simulink model "Copy_of_model"  (R2016b)
settings: Solver=FixedStepAuto  StartTime=0.0  StopTime=150  FixedStep=0.01  RelTol=1e-3
undefined symbols (not defined in the file or in its folder): DiscIntNeverNeededParam
libraries: dspsrcs4 x1
settings Model: Creator=Utente  LastModifiedBy=liana

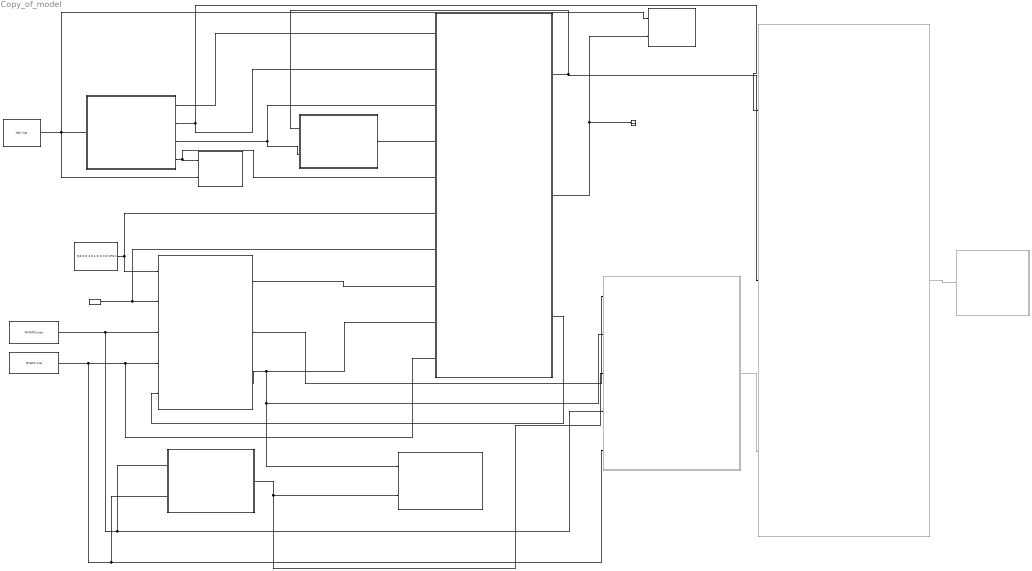
== system Copy_of_model ==
  Algebraic Transformation : Subsystem
  Attitude Observer : Subsystem
  Error position (AT) : Subsystem
  Error position (NLO) : Subsystem
  From File2 : FromFile  FileName=MYGYRO.mat  SampleTime=0.01
  From File3 : FromFile  FileName=MYACC.mat  SampleTime=0.01
  Gain computation : Subsystem
  Kalman - Bucy Filter : Subsystem  Commented=on
  Kp : Constant  Value=[10 0 0; 0 0.1 0; 0 0 0.1]*0.1  SampleTime=-1
  Mechanisation : Subsystem
  Scope : Scope
  Translational Motion Observer : Subsystem
  Vehicle position in NED : FromFile  FileName=NAV.mat
  angles error : Subsystem
  error : Subsystem  Commented=on
  sigma : Constant  Value=5  SampleTime=-1
  u computation : Subsystem  Commented=on
  wires:
  From File2/1 -> u computation/4(w_ib), Mechanisation/1(w_ib), Attitude Observer/3(w_ib)
  From File3/1 -> u computation/5(f_b), Mechanisation/2(f_b), Translational Motion Observer/10(f_b), Attitude Observer/4(f_b)
  Kp/1 -> Translational Motion Observer/6(K_p), Attitude Observer/1(Kp)
  sigma/1 -> Attitude Observer/2(sigma), Translational Motion Observer/7(sigma)
  Attitude Observer/1(J) -> Translational Motion Observer/8(J)
  Attitude Observer/3(R_nb_stim) -> angles error/1(R_nb_stim), u computation/2(R_nb_stim), Translational Motion Observer/9(R_nb_stim)
  Gain computation/1(K) -> Translational Motion Observer/4(K)
  Algebraic Transformation/3(C_dx) -> Gain computation/2(C_dx), Translational Motion Observer/3(C_dx)
  Translational Motion Observer/2(x_stim) -> Scope/1, Error position (NLO)/2(estimated)
  Vehicle position in NED/1 -> Error position (NLO)/1(true), Error position (AT)/2(true), Algebraic Transformation/1(p_n)
  Translational Motion Observer/3(f_n_stim) -> Attitude Observer/5(f_n_stim)
  Algebraic Transformation/4(x_at) -> Error position (AT)/1(estimated), Translational Motion Observer/5(Init)
  Mechanisation/1(R_nb) -> u computation/3(R_nb), angles error/2(R_nb)
  Algebraic Transformation/1(p_n_i) -> Translational Motion Observer/1(p_n_i)
  Translational Motion Observer/1(C_dx_NLO) -> Gain computation/1(C_dx_NLO), Kalman - Bucy Filter/2(C)
  Algebraic Transformation/2(delta) -> Translational Motion Observer/2(delta), Kalman - Bucy Filter/1(y)
  Attitude Observer/2(b_stim) -> u computation/1(b_stim)
  u computation/1(u) -> Kalman - Bucy Filter/3(U)
  Kalman - Bucy Filter/1(csi) -> error/1(csi)

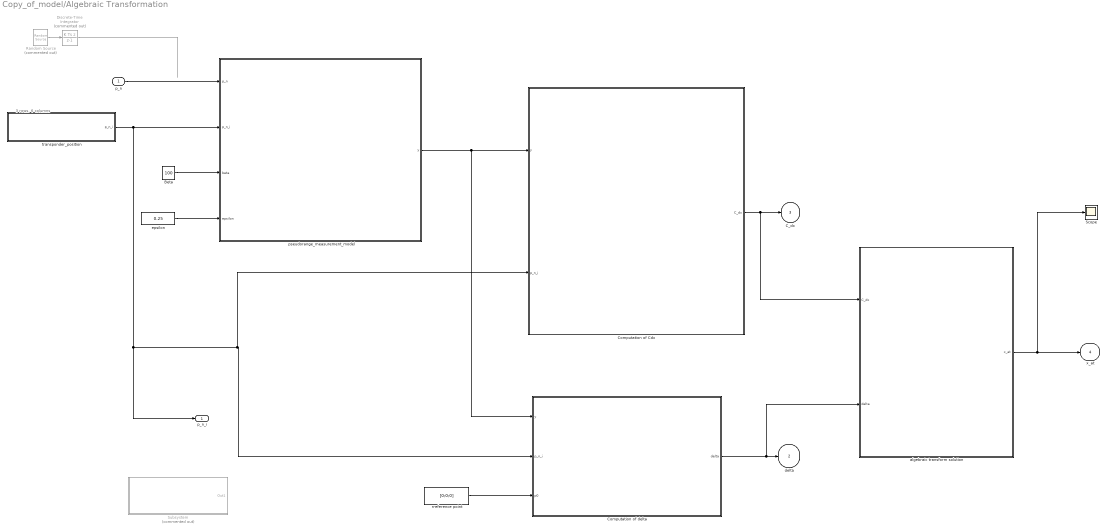
== system Copy_of_model/Algebraic Transformation ==
  note: 3 rows, 6 columns
  p_n : Inport
  Beta : Constant  Value=100
  Computation of Cdx : MATLAB Function  TreatAsAtomicUnit=on
  Computation of delta : MATLAB Function  TreatAsAtomicUnit=on
  Discrete-Time Integrator : DiscreteIntegrator  Commented=on  IntegratorMethod=Integration: Backward Euler  InitialConditionSetting=State (most efficient)  SampleTime=0.1  LimitOutput=on  UpperSaturationLimit=10  LowerSaturationLimit=-10  ICPrevOutput=DiscIntNeverNeededParam  ICPrevScaledInput=DiscIntNeverNeededParam
  Random Source : dspsrcs4/Random Source  Commented=on  SrcType=Gaussian  NormMethod=Ziggurat  CltLength=12  MinVal=0  MaxVal=1  MeanVal=[0;0;0]  VarVal=[1;1;1]*10  RepMode=Not repeatable  rawSeed=1  IsInherit=off  SampMode=Discrete  SampTime=0.1  SampFrame=1  DataType=Double  OutComplex=Real  OutputFrames=off
  Scope : Scope
  Subsystem : Subsystem  Commented=on
  algebraic transform solution : MATLAB Function  TreatAsAtomicUnit=on
  epsilon : Constant  Value=0.25
  pseudorange_measurement_model : MATLAB Function  TreatAsAtomicUnit=on
  rreference point : Constant  Value=[0;0;0]
  transponder_position : Subsystem
  p_n_i : Outport
  delta : Outport  Port=2
  C_dx : Outport  Port=3
  x_at : Outport  Port=4
  wires:
  Beta/1 -> pseudorange_measurement_model/3(beta)
  epsilon/1 -> pseudorange_measurement_model/4(epsilon)
  pseudorange_measurement_model/1(y) -> Computation of delta/1(y), Computation of Cdx/1(y)
  Computation of delta/1(delta) -> algebraic transform solution/2(delta), delta/1
  Computation of Cdx/1(C_dx) -> C_dx/1, algebraic transform solution/1(C_dx)
  rreference point/1 -> Computation of delta/3(p0)
  algebraic transform solution/1(x_at) -> Scope/1, x_at/1
  p_n/1 -> pseudorange_measurement_model/1(p_n)
  Discrete-Time Integrator/1 -> ?
  Random Source/1 -> Discrete-Time Integrator/1
  transponder_position/1(p_n_i) -> Computation of Cdx/2(p_n_i), Computation of delta/2(p_n_i), p_n_i/1, pseudorange_measurement_model/2(p_n_i)

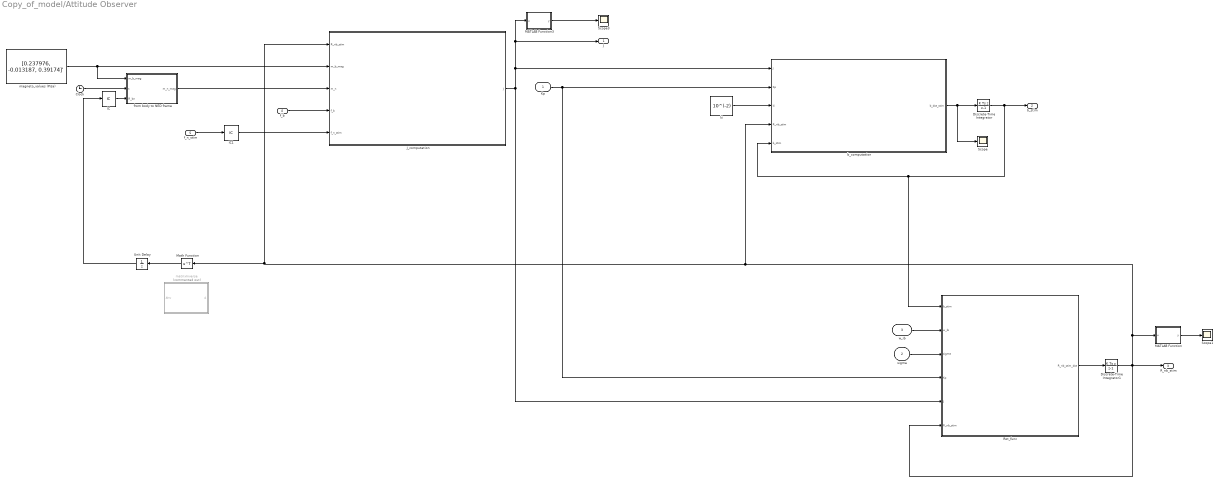
== system Copy_of_model/Attitude Observer ==
  Kp : Inport
  sigma : Inport  Port=2
  w_ib : Inport  Port=3
  f_b : Inport  Port=4
  f_n_stim : Inport  Port=5
  Clock : Clock
  Discrete-Time Integrator : DiscreteIntegrator  IntegratorMethod=Integration: Backward Euler  InitialConditionSetting=State (most efficient)  SampleTime=-1  ICPrevOutput=DiscIntNeverNeededParam  ICPrevScaledInput=DiscIntNeverNeededParam
  Discrete-Time Integrator1 : DiscreteIntegrator  IntegratorMethod=Integration: Backward Euler  InitialCondition=eye(3)  InitialConditionSetting=State (most efficient)  SampleTime=-1  ICPrevOutput=DiscIntNeverNeededParam  ICPrevScaledInput=DiscIntNeverNeededParam
  IC : InitialCondition  Value=eye(3)
  IC1 : InitialCondition  Value=[0;0;0]
  J_computation : Subsystem
  MATLAB Function : MATLAB Function  TreatAsAtomicUnit=on
  MATLAB Function3 : MATLAB Function  TreatAsAtomicUnit=on
  Math Function : Math  Operator=transpose  SaturateOnIntegerOverflow=on
  Rot_func : MATLAB Function  TreatAsAtomicUnit=on
  Scope : Scope
  Scope1 : Scope
  Scope3 : Scope
  Unit Delay : UnitDelay  SampleTime=-1
  b_computation : MATLAB Function  TreatAsAtomicUnit=on
  from body to NED frame : MATLAB Function  TreatAsAtomicUnit=on
  ki : Constant  Value=10^(-2)  SampleTime=-1
  magneto_values (Pisa) : Constant  Value=[0.237976, -0.013187, 0.39174]'
  matrixInverse : MATLAB Function  Commented=on  TreatAsAtomicUnit=on
  J : Outport
  b_stim : Outport  Port=2
  R_nb_stim : Outport  Port=3
  wires:
  magneto_values (Pisa)/1 -> from body to NED frame/1(m_b_mag), J_computation/2(m_b_mag)
  from body to NED frame/1(m_n_mag) -> J_computation/3(m_n)
  f_b/1 -> J_computation/4(f_b)
  J_computation/1(J) -> MATLAB Function3/1(u), J/1, b_computation/1(J), Rot_func/5(J)
  Kp/1 -> Rot_func/4(Kp), b_computation/2(Kp)
  ki/1 -> b_computation/3(ki)
  sigma/1 -> Rot_func/3(sigma)
  w_ib/1 -> Rot_func/2(w_ib)
  Clock/1 -> from body to NED frame/2(t)
  b_computation/1(b_dot_stim) -> Scope/1, Discrete-Time Integrator/1
  MATLAB Function/1(y) -> Scope1/1
  MATLAB Function3/1(y) -> Scope3/1
  f_n_stim/1 -> IC1/1
  Rot_func/1(R_nb_stim_dot) -> Discrete-Time Integrator1/1
  Discrete-Time Integrator/1 -> b_stim/1, Rot_func/1(b_stim), b_computation/5(b_stim)
  Discrete-Time Integrator1/1 -> R_nb_stim/1, Rot_func/6(R_nb_stim), Math Function/1, J_computation/1(R_nb_stim), b_computation/4(R_nb_stim), MATLAB Function/1(u)
  IC/1 -> from body to NED frame/3(R_bn)
  Math Function/1 -> Unit Delay/1
  Unit Delay/1 -> IC/1
  IC1/1 -> J_computation/5(f_n_stim)

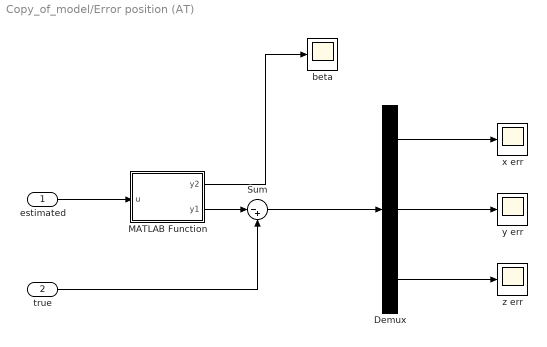
== system Copy_of_model/Error position (AT) ==
  estimated : Inport
  true : Inport  Port=2
  Demux : Demux  Outputs=3
  MATLAB Function : MATLAB Function  TreatAsAtomicUnit=on
  Sum : Sum  Inputs=|-+
  beta : Scope
  x err : Scope
  y err : Scope
  z err : Scope
  wires:
  estimated/1 -> MATLAB Function/1(u)
  MATLAB Function/2(y1) -> Sum/1
  true/1 -> Sum/2
  Sum/1 -> Demux/1
  Demux/1 -> x err/1
  Demux/2 -> y err/1
  Demux/3 -> z err/1
  MATLAB Function/1(y2) -> beta/1

== system Copy_of_model/Error position (NLO) ==
  true : Inport
  estimated : Inport  Port=2
  Demux : Demux  Outputs=3
  MATLAB Function : MATLAB Function  TreatAsAtomicUnit=on
  Sum : Sum  Inputs=|-+
  x err : Scope
  y err : Scope
  z err : Scope
  wires:
  estimated/1 -> MATLAB Function/1(u)
  MATLAB Function/1(y) -> Sum/1
  true/1 -> Sum/2
  Sum/1 -> Demux/1
  Demux/1 -> x err/1
  Demux/2 -> y err/1
  Demux/3 -> z err/1

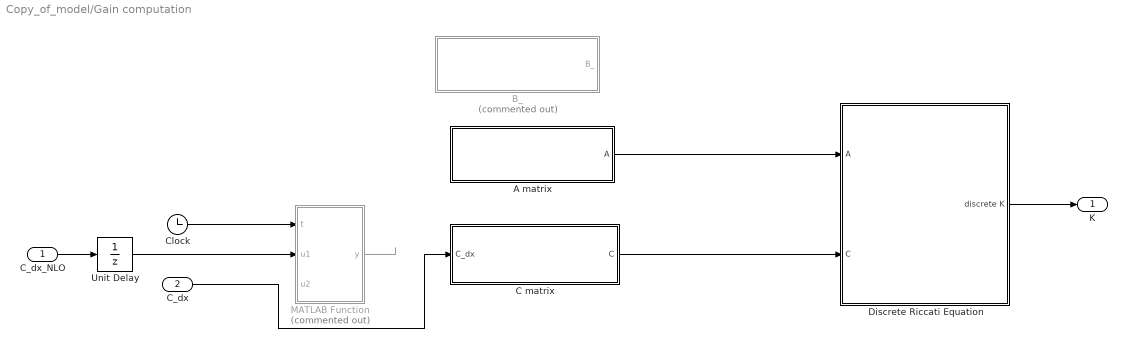
== system Copy_of_model/Gain computation ==
  C_dx_NLO : Inport
  C_dx : Inport  Port=2
  A matrix : MATLAB Function  TreatAsAtomicUnit=on
  B_ : MATLAB Function  Commented=on  TreatAsAtomicUnit=on
  C matrix : MATLAB Function  TreatAsAtomicUnit=on
  Clock : Clock
  Discrete Riccati Equation : Subsystem
  MATLAB Function : MATLAB Function  Commented=on  TreatAsAtomicUnit=on
  Unit Delay : UnitDelay  SampleTime=-1
  K : Outport
  wires:
  C matrix/1(C) -> Discrete Riccati Equation/2(C)
  A matrix/1(A) -> Discrete Riccati Equation/1("A ")
  C_dx/1 -> C matrix/1(C_dx)
  Discrete Riccati Equation/1(discrete K) -> K/1
  Clock/1 -> MATLAB Function/1(t)
  C_dx_NLO/1 -> Unit Delay/1
  MATLAB Function/1(y) -> ?
  Unit Delay/1 -> MATLAB Function/2(u1)

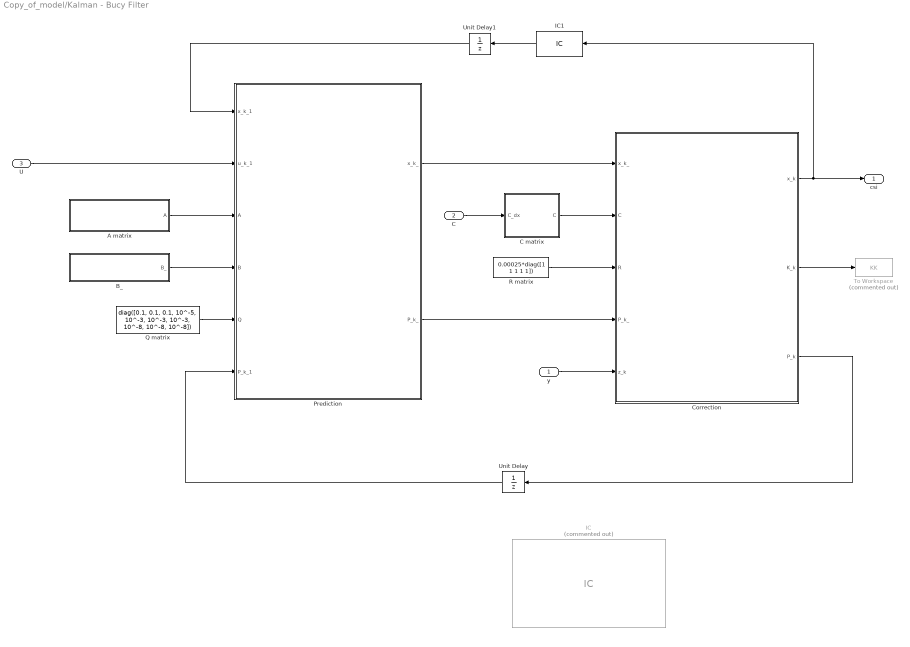
== system Copy_of_model/Kalman - Bucy Filter ==
  y : Inport
  C : Inport  Port=2
  U : Inport  Port=3
  A matrix : MATLAB Function  TreatAsAtomicUnit=on
  B_ : MATLAB Function  TreatAsAtomicUnit=on
  C matrix : MATLAB Function  TreatAsAtomicUnit=on
  Correction : MATLAB Function  TreatAsAtomicUnit=on
  IC : InitialCondition  Commented=on  Value=diag([3*(10^3),3*(10^3),3*(10^3),3*(10^3),10,10,10,0.01,0.01,0.01])
  IC1 : InitialCondition  Value=zeros(10,1)
  Prediction : MATLAB Function  TreatAsAtomicUnit=on
  Q matrix : Constant  Value=diag([0.1, 0.1, 0.1, 10^-5, 10^-3, 10^-3, 10^-3, 10^-8, 10^-8, 10^-8])
  R matrix : Constant  Value=0.00025*diag([1 1 1 1 1])
  To Workspace : ToWorkspace  Commented=on  VariableName=KK  SaveFormat=Timeseries  SampleTime=-1
  Unit Delay : UnitDelay  InitialCondition=eye(10)*10  SampleTime=-1
  Unit Delay1 : UnitDelay  SampleTime=-1
  csi : Outport
  wires:
  Prediction/2(P_k_) -> Correction/4(P_k_)
  Prediction/1(x_k_) -> Correction/1(x_k_)
  Correction/1(x_k) -> csi/1, IC1/1
  A matrix/1(A) -> Prediction/3(A)
  C matrix/1(C) -> Correction/2(C)
  B_/1(B_) -> Prediction/4(B)
  U/1 -> Prediction/2(u_k_1)
  R matrix/1 -> Correction/3(R)
  Correction/3(P_k) -> Unit Delay/1
  Unit Delay/1 -> Prediction/6(P_k_1)
  Correction/2(K_k) -> To Workspace/1
  Unit Delay1/1 -> Prediction/1(x_k_1)
  y/1 -> Correction/5(z_k)
  Q matrix/1 -> Prediction/5(Q)
  IC1/1 -> Unit Delay1/1
  C/1 -> C matrix/1(C_dx)

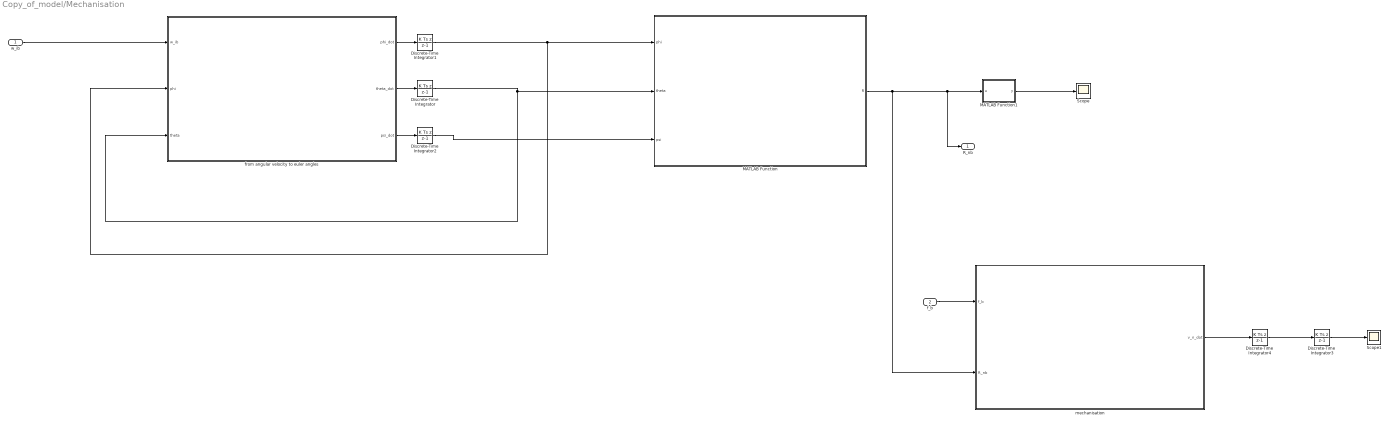
== system Copy_of_model/Mechanisation ==
  w_ib : Inport
  f_b : Inport  Port=2
  Discrete-Time Integrator{,1..4} (5 alike) : DiscreteIntegrator  IntegratorMethod=Integration: Backward Euler  InitialConditionSetting=State (most efficient)  SampleTime=-1  ICPrevOutput=DiscIntNeverNeededParam  ICPrevScaledInput=DiscIntNeverNeededParam
  MATLAB Function : MATLAB Function  TreatAsAtomicUnit=on
  MATLAB Function1 : MATLAB Function  TreatAsAtomicUnit=on
  Scope : Scope
  Scope1 : Scope
  from angular velocity to euler angles : MATLAB Function  TreatAsAtomicUnit=on
  mechanisation : MATLAB Function  TreatAsAtomicUnit=on
  R_nb : Outport
  wires:
  w_ib/1 -> from angular velocity to euler angles/1(w_ib)
  from angular velocity to euler angles/1(phi_dot) -> Discrete-Time Integrator1/1
  from angular velocity to euler angles/2(theta_dot) -> Discrete-Time Integrator/1
  from angular velocity to euler angles/3(psi_dot) -> Discrete-Time Integrator2/1
  MATLAB Function/1(R) -> mechanisation/2(R_nb), R_nb/1, MATLAB Function1/1(u)
  MATLAB Function1/1(y) -> Scope/1
  f_b/1 -> mechanisation/1(f_b)
  Discrete-Time Integrator4/1 -> Discrete-Time Integrator3/1
  Discrete-Time Integrator3/1 -> Scope1/1
  mechanisation/1(v_n_dot) -> Discrete-Time Integrator4/1
  Discrete-Time Integrator/1 -> from angular velocity to euler angles/3(theta), MATLAB Function/2(theta)
  Discrete-Time Integrator2/1 -> MATLAB Function/3(psi)
  Discrete-Time Integrator1/1 -> from angular velocity to euler angles/2(phi), MATLAB Function/1(phi)

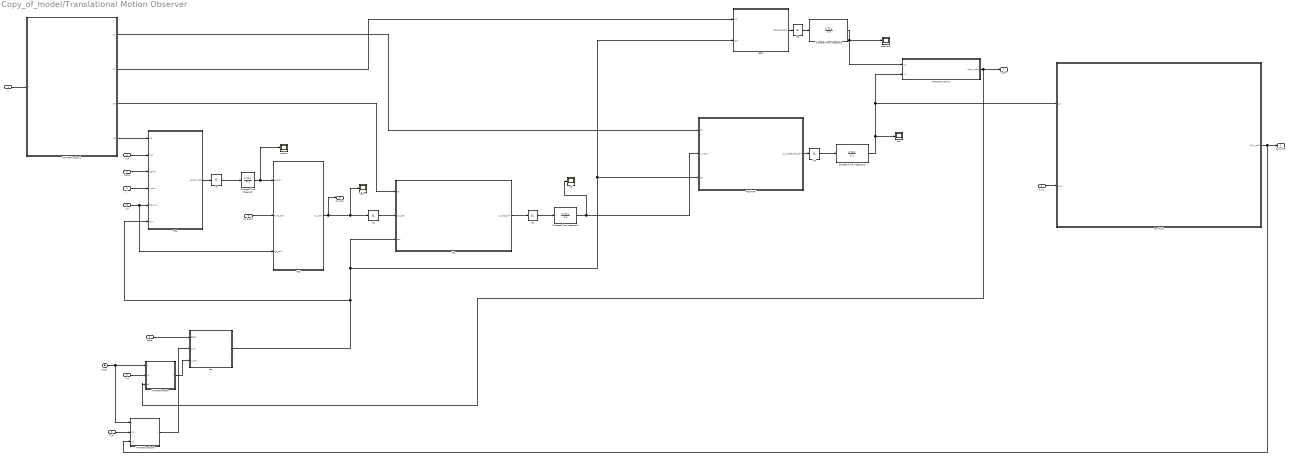
== system Copy_of_model/Translational Motion Observer ==
  p_n_i : Inport
  delta : Inport  Port=2
  C_dx : Inport  Port=3
  K : Inport  Port=4
  Init : Inport  Port=5
  K_p : Inport  Port=6
  sigma : Inport  Port=7
  J : Inport  Port=8
  R_nb_stim : Inport  Port=9
  f_b : Inport  Port=10
  ACC : MATLAB Function  TreatAsAtomicUnit=on
  BETA : MATLAB Function  TreatAsAtomicUnit=on
  Clock : Clock
      settings: Decimation=2
  Discrete-Time Integrator : DiscreteIntegrator  IntegratorMethod=Integration: Backward Euler  InitialCondition=[0;0;0]  InitialConditionSetting=State (most efficient)  SampleTime=-1  ICPrevOutput=DiscIntNeverNeededParam  ICPrevScaledInput=DiscIntNeverNeededParam
  Discrete-Time Integrator1 : DiscreteIntegrator  IntegratorMethod=Integration: Backward Euler  InitialCondition=[0;0;0]  InitialConditionSetting=State (most efficient)  SampleTime=-1  ICPrevOutput=DiscIntNeverNeededParam  ICPrevScaledInput=DiscIntNeverNeededParam
  Discrete-Time Integrator2 : DiscreteIntegrator  IntegratorMethod=Integration: Backward Euler  InitialCondition=[10;0;0]  InitialConditionSetting=State (most efficient)  SampleTime=-1  ICPrevOutput=DiscIntNeverNeededParam  ICPrevScaledInput=DiscIntNeverNeededParam
  Discrete-Time Integrator3 : DiscreteIntegrator  IntegratorMethod=Integration: Backward Euler  InitialConditionSetting=State (most efficient)  SampleTime=-1  ICPrevOutput=DiscIntNeverNeededParam  ICPrevScaledInput=DiscIntNeverNeededParam
  EPS : MATLAB Function  TreatAsAtomicUnit=on
  IC{,1..2,4} (4 alike) : InitialCondition  Value=[0;0;0]
  IC3 : InitialCondition  Value=0
  MATLAB Function : MATLAB Function  TreatAsAtomicUnit=on
  MATLAB Function1 : MATLAB Function  TreatAsAtomicUnit=on
  MATLAB Function2 : MATLAB Function  TreatAsAtomicUnit=on
  MATLAB Function3 : MATLAB Function  TreatAsAtomicUnit=on
  POSITION : MATLAB Function  TreatAsAtomicUnit=on
  VEL : MATLAB Function  TreatAsAtomicUnit=on
  beta stim : Scope
  corr : MATLAB Function  TreatAsAtomicUnit=on
  epsilon : Scope
  f_stim : Scope
  new C_dx : Subsystem
  pos : Scope
  vel : Scope
  C_dx_NLO : Outport
  x_stim : Outport  Port=2
  f_n_stim : Outport  Port=3
  wires:
  EPS/1(epsilon_dot) -> IC/1
  Discrete-Time Integrator/1 -> epsilon/1, ACC/1(epsilon)
  MATLAB Function1/4(K4) -> EPS/1(K4)
  MATLAB Function1/1(K1) -> POSITION/1(K1)
  MATLAB Function1/3(K3) -> VEL/1(K3)
  MATLAB Function1/2(K2) -> BETA/1(K2)
  BETA/1(beta_dot_stim) -> IC3/1
  POSITION/1(p_n_delta_dot_stim) -> IC4/1
  VEL/1(v_n_dot_stim) -> IC2/1
  MATLAB Function2/1(new_x_stim) -> x_stim/1, MATLAB Function/3(u2)
  K/1 -> MATLAB Function1/1(K)
  K_p/1 -> EPS/2(K_p)
  sigma/1 -> EPS/3(sigma)
  J/1 -> EPS/4(J_stim)
  f_b/1 -> ACC/3(f_b_imu), EPS/5(f_b_imu)
  R_nb_stim/1 -> ACC/2(R_nb_stim)
  C_dx/1 -> MATLAB Function3/2(u1)
  delta/1 -> corr/1(delta)
  Init/1 -> MATLAB Function/2(u1)
  MATLAB Function/1(y) -> corr/3(x_stim)
  Clock/1 -> MATLAB Function3/1(t), MATLAB Function/1(t)
  ACC/1(f_n_stim) -> f_n_stim/1, IC1/1, f_stim/1
  IC/1 -> Discrete-Time Integrator/1
  IC1/1 -> VEL/2(f_n_stim)
  Discrete-Time Integrator1/1 -> vel/1, POSITION/2(v_n_stim)
  Discrete-Time Integrator3/1 -> beta stim/1, MATLAB Function2/1(u2)
  Discrete-Time Integrator2/1 -> pos/1, new C_dx/1(p_n), MATLAB Function2/2(u1)
  IC3/1 -> Discrete-Time Integrator3/1
  IC4/1 -> Discrete-Time Integrator2/1
  IC2/1 -> Discrete-Time Integrator1/1
  new C_dx/1(C_dx_NLO) -> MATLAB Function3/3(u2), C_dx_NLO/1
  MATLAB Function3/1(y) -> corr/2(C_dx)
  corr/1(y) -> BETA/2(corr), POSITION/3(corr), VEL/3(corr), EPS/6(corr)
  p_n_i/1 -> new C_dx/2(p_n_i)

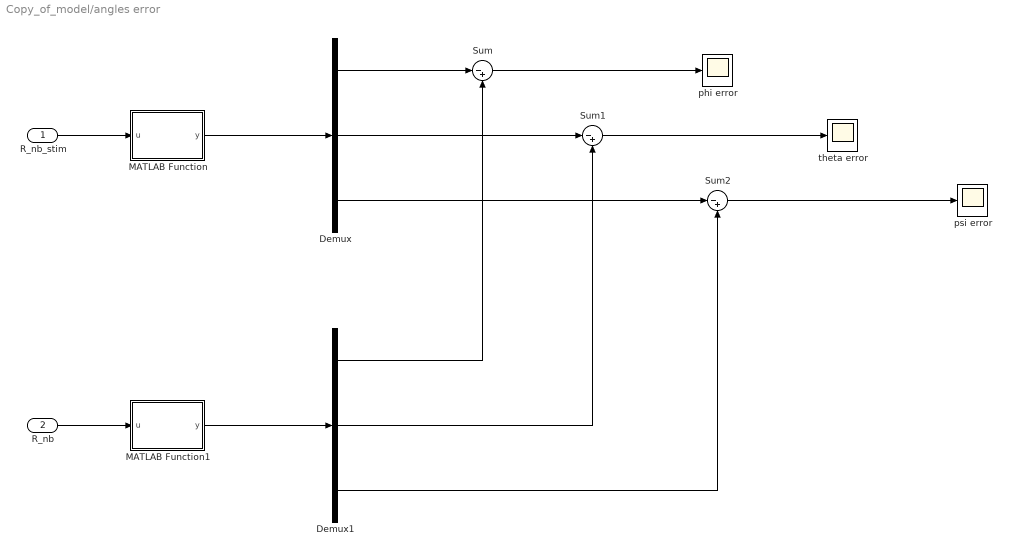
== system Copy_of_model/angles error ==
  R_nb_stim : Inport
  R_nb : Inport  Port=2
  Demux : Demux  Outputs=3
  Demux1 : Demux  Outputs=3
  MATLAB Function : MATLAB Function  TreatAsAtomicUnit=on
  MATLAB Function1 : MATLAB Function  TreatAsAtomicUnit=on
  Sum : Sum  Inputs=|-+
  Sum1 : Sum  Inputs=|-+
  Sum2 : Sum  Inputs=|-+
  phi error : Scope
  psi error : Scope
  theta error : Scope
  wires:
  R_nb_stim/1 -> MATLAB Function/1(u)
  R_nb/1 -> MATLAB Function1/1(u)
  MATLAB Function/1(y) -> Demux/1
  MATLAB Function1/1(y) -> Demux1/1
  Demux/1 -> Sum/1
  Demux/2 -> Sum1/1
  Demux/3 -> Sum2/1
  Demux1/1 -> Sum/2
  Demux1/2 -> Sum1/2
  Demux1/3 -> Sum2/2
  Sum/1 -> phi error/1
  Sum1/1 -> theta error/1
  Sum2/1 -> psi error/1

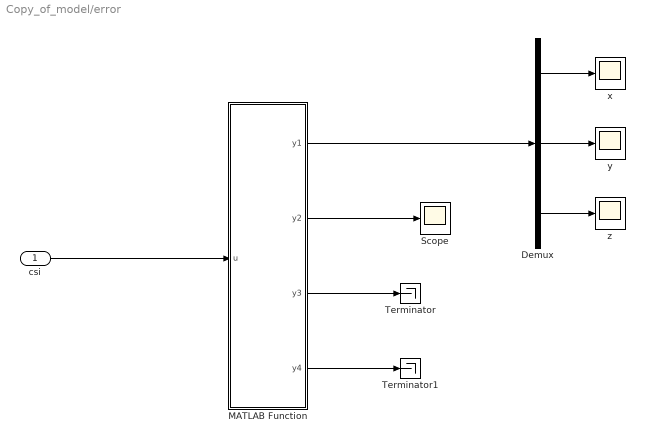
== system Copy_of_model/error ==
  csi : Inport
  Demux : Demux  Outputs=3
  MATLAB Function : MATLAB Function  TreatAsAtomicUnit=on
  Scope : Scope
  Terminator : Terminator
  Terminator1 : Terminator
  x : Scope
  y : Scope
  z : Scope
  wires:
  csi/1 -> MATLAB Function/1(u)
  MATLAB Function/3(y3) -> Terminator/1
  MATLAB Function/4(y4) -> Terminator1/1
  MATLAB Function/1(y1) -> Demux/1
  MATLAB Function/2(y2) -> Scope/1
  Demux/1 -> x/1
  Demux/2 -> y/1
  Demux/3 -> z/1

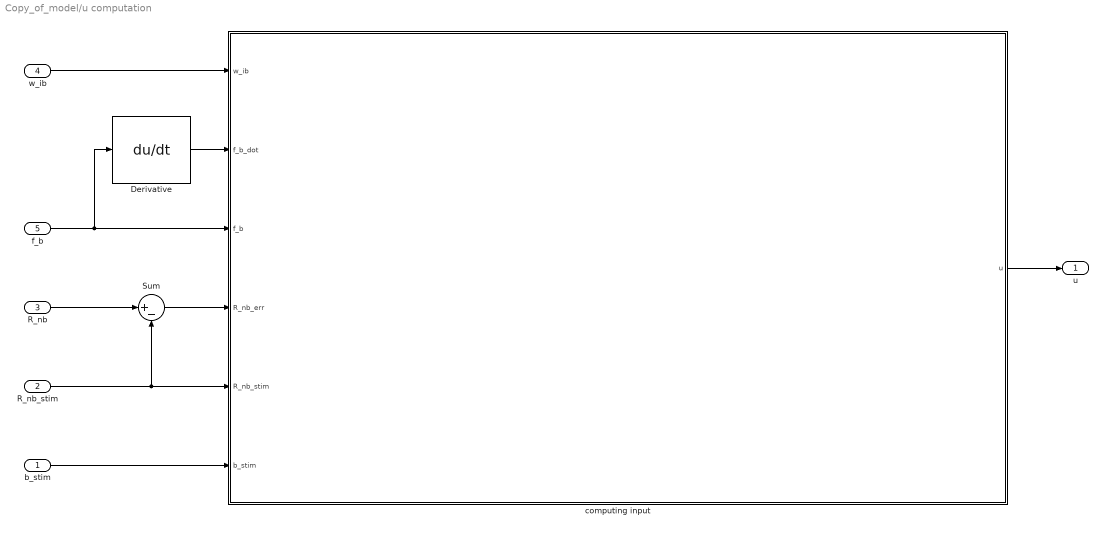
== system Copy_of_model/u computation ==
  b_stim : Inport
  R_nb_stim : Inport  Port=2
  R_nb : Inport  Port=3
  w_ib : Inport  Port=4
  f_b : Inport  Port=5
  Derivative : Derivative
  Sum : Sum  Inputs=|+-
  computing input : MATLAB Function  TreatAsAtomicUnit=on
  u : Outport
  wires:
  Derivative/1 -> computing input/2(f_b_dot)
  computing input/1(u) -> u/1
  b_stim/1 -> computing input/6(b_stim)
  Sum/1 -> computing input/4(R_nb_err)
  R_nb_stim/1 -> Sum/2, computing input/5(R_nb_stim)
  R_nb/1 -> Sum/1
  f_b/1 -> Derivative/1, computing input/3(f_b)
  w_ib/1 -> computing input/1(w_ib)

== system Copy_of_model/Algebraic Transformation/Subsystem ==
  Matrix Concatenate (transponders positions) : Concatenate  NumInputs=6  Mode=Multidimensional array  ConcatenateDimension=2
  p_n_1 : Constant  Value=[800; 110; 0]
  p_n_2 : Constant  Value=[500; 180; 1]
  p_n_3 : Constant  Value=[1500; 200; 3]
  p_n_4 : Constant  Value=[950; 250; 10]
  p_n_5 : Constant  Value=[750; 150; 7]
  p_n_6 : Constant  Value=[300; 20; 9]
  Out1 : Outport
  wires:
  Matrix Concatenate (transponders positions)/1 -> Out1/1
  p_n_5/1 -> Matrix Concatenate (transponders positions)/5
  p_n_1/1 -> Matrix Concatenate (transponders positions)/1
  p_n_3/1 -> Matrix Concatenate (transponders positions)/3
  p_n_4/1 -> Matrix Concatenate (transponders positions)/4
  p_n_6/1 -> Matrix Concatenate (transponders positions)/6
  p_n_2/1 -> Matrix Concatenate (transponders positions)/2

== system Copy_of_model/Algebraic Transformation/transponder_position ==
  Matrix Concatenate (transponders positions) : Concatenate  NumInputs=6  Mode=Multidimensional array  ConcatenateDimension=2
  p_n_1 : Constant  Value=[750, 0, 10]
  p_n_2 : Constant  Value=[0, 1000, 15]
  p_n_3 : Constant  Value=[0, 700, 10]
  p_n_4 : Constant  Value=[1500, 0, 20]
  p_n_6 : Constant  Value=[0, 600, 10]
  p_n_7 : Constant  Value=[1000, 0, 100]
  p_n_i : Outport
  wires:
  p_n_4/1 -> Matrix Concatenate (transponders positions)/4
  p_n_7/1 -> Matrix Concatenate (transponders positions)/5
  p_n_3/1 -> Matrix Concatenate (transponders positions)/6
  Matrix Concatenate (transponders positions)/1 -> p_n_i/1
  p_n_1/1 -> Matrix Concatenate (transponders positions)/1
  p_n_2/1 -> Matrix Concatenate (transponders positions)/2
  p_n_6/1 -> Matrix Concatenate (transponders positions)/3

== system Copy_of_model/Attitude Observer/J_computation ==
  R_nb_stim : Inport
  m_b_mag : Inport  Port=2
  m_n : Inport  Port=3
  f_b : Inport  Port=4
  f_n_stim : Inport  Port=5  PortDimensions=[3,1]
  q computation : MATLAB Function  TreatAsAtomicUnit=on
  J : Outport
  wires:
  m_n/1 -> q computation/2(m_n)
  f_n_stim/1 -> q computation/4(f_n_stim)
  m_b_mag/1 -> q computation/1(m_b_mag)
  f_b/1 -> q computation/3(f_b)
  q computation/1(J) -> J/1
  R_nb_stim/1 -> q computation/5(R_nb_stim)

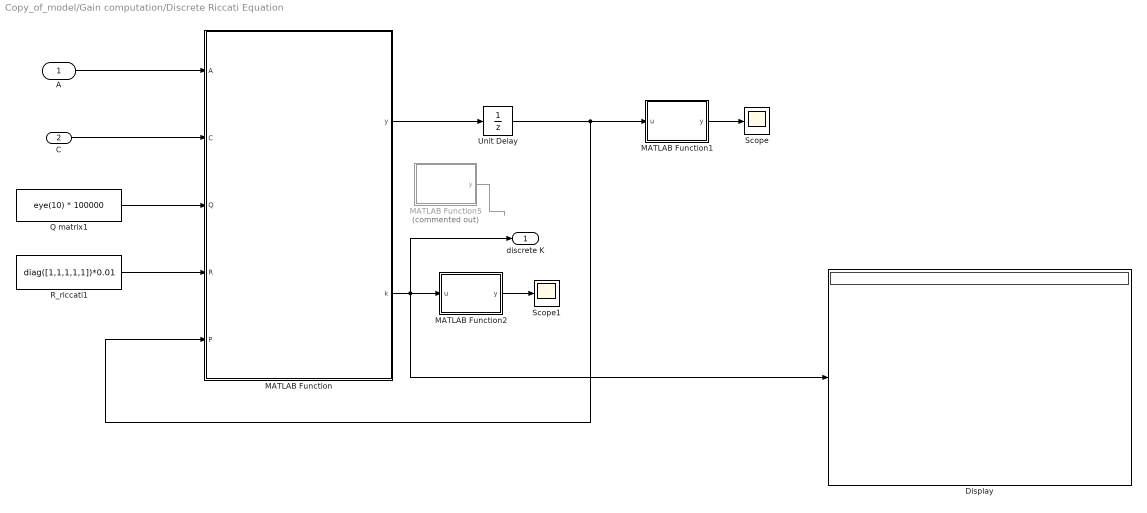
== system Copy_of_model/Gain computation/Discrete Riccati Equation ==
  "A " : Inport
  C : Inport  Port=2
  Display : Display
  MATLAB Function : MATLAB Function  TreatAsAtomicUnit=on
  MATLAB Function1 : MATLAB Function  TreatAsAtomicUnit=on
  MATLAB Function2 : MATLAB Function  TreatAsAtomicUnit=on
  MATLAB Function5 : MATLAB Function  Commented=on  TreatAsAtomicUnit=on
  Q matrix1 : Constant  Value=eye(10) * 100000  SampleTime=-1
  R_riccati1 : Constant  Value=diag([1,1,1,1,1])*0.01  VectorParams1D=off  SampleTime=-1
  Scope : Scope
  Scope1 : Scope
  Unit Delay : UnitDelay  InitialCondition=eye(10)*100  SampleTime=-1
  discrete K : Outport
  wires:
  C/1 -> MATLAB Function/2(C)
  Q matrix1/1 -> MATLAB Function/3(Q)
  R_riccati1/1 -> MATLAB Function/4(R)
  Unit Delay/1 -> MATLAB Function1/1(u), MATLAB Function/5(P)
  MATLAB Function1/1(y) -> Scope/1
  MATLAB Function2/1(y) -> Scope1/1
  MATLAB Function/1(y) -> Unit Delay/1
  "A "/1 -> MATLAB Function/1(A)
  MATLAB Function/2(k) -> discrete K/1, Display/1, MATLAB Function2/1(u)
  MATLAB Function5/1(y) -> ?

== system Copy_of_model/Translational Motion Observer/new C_dx ==
  p_n : Inport
  p_n_i : Inport  Port=2
  Computation of Cdx : MATLAB Function  TreatAsAtomicUnit=on
  pseudorange_measurement_model : MATLAB Function  TreatAsAtomicUnit=on
  C_dx_NLO : Outport
  wires:
  p_n_i/1 -> Computation of Cdx/2(p_n_i), pseudorange_measurement_model/2(p_n_i)
  pseudorange_measurement_model/1(y) -> Computation of Cdx/1(y)
  Computation of Cdx/1(C_dx) -> C_dx_NLO/1
  p_n/1 -> pseudorange_measurement_model/1(p_n)

== matlab function Copy_of_model/Attitude Observer/J_computation/q computation ==
  data: m_b_mag input; m_n input; f_b input; f_n_stim input size=3; J output; R_nb_stim input size=[3,3]
function J  = qEfunc(m_b_mag, m_n, f_b, f_n_stim, R_nb_stim)

g_n = [0.1 0.1 0.1]';   % gravity compensated

q1_b = m_b_mag/norm(m_b_mag,2);
q2_b = f_b/norm(g_n,2);

q1_n = m_n/norm(m_n,2);
q2_n = f_n_stim/norm(g_n,2);

E_b = [q1_b, skew(q1_b)*q2_b, (skew(q1_b)*skew(q1_b))*q2_b];
E_n = [q1_n, skew(q1_n)*q2_n, (skew(q1_n)*skew(q1_n))*q2_n];

J = (E_n - R_nb_stim * E_b) * (E_b');

end

== matlab function Copy_of_model/Error position (AT)/MATLAB Function ==
  data: y2 output; u input; y1 output
function [y2,y1] = fcn(u)

y1 = u(1:3,1);
y2 = u(4,1);

== matlab function Copy_of_model/Translational Motion Observer/MATLAB Function ==
  data: t input; y output; u1 input; u2 input
function y = fcn(t,u1,u2)

if t == 0
    y = u1;
else
    y = u2;
end

== matlab function Copy_of_model/Error position (NLO)/MATLAB Function ==
  data: u input; y output
function y = fcn(u)

y = u(1:3,1);

== matlab function Copy_of_model/angles error/MATLAB Function ==
  data: u input; y output
function y = fcn(u)

y = rotm2eul(u,'ZYX');

== matlab function Copy_of_model/angles error/MATLAB Function1 ==
  data: u input; y output
function y = fcn(u)

y = rotm2eul(u,'ZYX');

== matlab function Copy_of_model/Attitude Observer/b_computation ==
  data: J input; b_dot_stim output size=3; Kp input; ki input; R_nb_stim input; b_stim input
function b_dot_stim  = b_dot_stim_func(J, Kp, ki, R_nb_stim, b_stim)

SAT = sat(R_nb_stim)';

PA = pa( SAT * Kp * J);

VEX = vexfunc(PA);

b_dot_stim = Proj(b_stim , -ki * VEX);

end

== matlab function Copy_of_model/Translational Motion Observer/new C_dx/Computation of Cdx ==
  data: y input; p_n_i input; C_dx output size=[5,4]
function C_dx  = C_dx_func(y,p_n_i)

    [row,col] = size(p_n_i);
    [row_,col_] = size(y);

    % taking last transponder position
    p_m = p_n_i(:,col);
    
    % col is the number of transponders
    
    % taking last pseudorange measurement
    y_m = y(row_);
    
    %row vector, 3 stands for x,y,z
    p_ = zeros(col-1,3); 
    y_ = zeros(col-1,1);
    
    for i = 1:1:(col-1)
    
        p_(i,:) = (p_m - p_n_i(:,i))';
        
        y_(i,1) = y(i,1) - y_m;
        
    end
    
    C_dx = [p_, y_];

end

== matlab function Copy_of_model/Algebraic Transformation/Computation of Cdx ==
  data: y input; p_n_i input; C_dx output size=[5,4]
function C_dx  = C_dx_func(y,p_n_i)

    [row,col] = size(p_n_i);
    [row_,col_] = size(y);

    % taking last transponder position
    p_m = p_n_i(:,col);
    
    % col is the number of transponders
    
    % taking last pseudorange measurement
    y_m = y(row_);
    
    %row vector, 3 stands for x,y,z
    p_ = zeros(col-1,3); 
    y_ = zeros(col-1,1);
    
    for i = 1:1:(col-1)
    
        p_(i,:) = (p_m - p_n_i(:,i))';
        
        y_(i,1) = y(i,1) - y_m;
        
    end
    
    C_dx = [p_, y_];

end

== matlab function Copy_of_model/Algebraic Transformation/Computation of delta ==
  data: y input; delta output size=5; p_n_i input; p0 input
function delta = delta_func(y, p_n_i, p0)
    
    % col is the number of transponders
    [row,col] = size(p_n_i);
    %[row_,col_] = size(y);
    
    % line of sight between transponders and reference point
    p_los = zeros(row,col);
    
    for i = 1:1:col
       p_los(:,i) = p_n_i(:,i) - p0;
    end
    
    % useful variable
    z = zeros(col,1);
    
    for i = 1:1:col
        z(i,1)= ( (y(i,1)^2) - norm(p_los(:,i),2)^2 );
    end
    
    % computing delta
    delta = zeros(col-1,1);
    % last value of z
    z_m = z(col,1);
    
    for i=1:1:(col-1)
        delta(i,1) = z(i,1) - z_m;
    end
    
end

== matlab function Copy_of_model/Translational Motion Observer/new C_dx/pseudorange_measurement_model ==
  data: p_n input; y output size=[6,1]; p_n_i input
function y = pseudorange_mea_model(p_n, p_n_i)
  
  [r,c] = size(p_n_i);
  
  y = zeros(c,1);

  for i=1:1:c
      
      rho = norm(p_n - p_n_i(:,i),2);   % eq. 7
      
      y(i,1) = rho;      % eq. 8 

  end
      
end

== matlab function Copy_of_model/Gain computation/MATLAB Function ==
  data: t input; y output; u1 input; u2 input
function y = fcn(t,u1,u2)

if t==0
    y = u2;
else
    y = u1;
end

== matlab function Copy_of_model/Translational Motion Observer/MATLAB Function3 ==
  data: t input; y output; u1 input; u2 input
function y = fcn(t,u1,u2)

if t == 0
    y = u1;
else
    y = u2;
end

== matlab function Copy_of_model/Attitude Observer/Rot_func ==
  data: b_stim input; R_nb_stim_dot output; w_ib input; sigma input; Kp input; J input; R_nb_stim input
function R_nb_stim_dot  = rot_func(b_stim,w_ib,sigma,Kp,J,R_nb_stim) 

Skew = skew(w_ib - b_stim);

R_nb_stim_dot = R_nb_stim * Skew + sigma * Kp * J;

== matlab function Copy_of_model/Kalman - Bucy Filter/Correction ==
  data: x_k_ input; C input; R input size=[5,5]; P_k_ input size=[10,10]; z_k input; x_k output; K_k output size=[10,5]; P_k output
function [x_k,K_k, P_k]  = correction(x_k_ , C, R, P_k_ ,z_k)

    n = size(P_k_);
    
    K_k = zeros(10,5);
   
    
    K_k = P_k_ * C' * pinv(C * P_k_ * C' + R);
    
    x_k = x_k_ + K_k * (z_k - C * x_k_);
    
    P_k = (eye(n) - K_k * C) * P_k_;

end

== matlab function Copy_of_model/Kalman - Bucy Filter/Prediction ==
  data: x_k_1 input size=[10, 1]; u_k_1 input; A input; B input; Q input; P_k_1 input size=[10,10]; x_k_ output; P_k_ output
function [x_k_, P_k_] = prediction(x_k_1, u_k_1, A, B, Q, P_k_1)

    
%     x_k_ = (A - K*C) * x_k_1 + B * u_k_1;
%     
%     P_k_ = (A-K*C) * P_k_1 * (A-K*C)' + Q;
    
    
    x_k_ = A * x_k_1 + B * u_k_1;
    
    P_k_ = A * P_k_1 * A' + Q;

end

== matlab function Copy_of_model/Kalman - Bucy Filter/A matrix ==
  data: A output
function A = A()

 A = zeros(10);

 A(1:3,5:7) = eye(3);
 A(5:7,8:10) = eye(3);
 
end

== matlab function Copy_of_model/Gain computation/A matrix ==
  data: A output
function A = A()

 A = zeros(10);

 A(1:3,5:7) = eye(3);
 A(5:7,8:10) = eye(3);
 
end

== matlab function Copy_of_model/Gain computation/C matrix ==
  data: C output; C_dx input
function C = Cfunc(C_dx)

   row = size(C_dx,1); 

   C1 = zeros(row,6);

 C = [2*C_dx C1];
 
 
end

== matlab function Copy_of_model/Gain computation/B_ ==
  data: B_ output
function B_ = B()

 B_ = zeros(10,3);

 B_(8:10,1:3) = eye(3);
end

== matlab function Copy_of_model/Kalman - Bucy Filter/B_ ==
  data: B_ output
function B_ = B()

 B_ = zeros(10,3);

 B_(8:10,1:3) = eye(3);
end

== matlab function Copy_of_model/Algebraic Transformation/pseudorange_measurement_model ==
  data: p_n input; y output size=[6,1]; p_n_i input; beta input; epsilon input
function y = pseudorange_mea_model(p_n, p_n_i, beta, epsilon)
  
  [r,c] = size(p_n_i);
  
  y = zeros(c,1);

  for i=1:1:c
      
      rho = norm(p_n - p_n_i(:,i),2);   % eq. 7
      
      y(i,1) = rho + beta + epsilon;      % eq. 8 

  end
      
end

== matlab function Copy_of_model/u computation/computing input ==
  data: w_ib input; f_b_dot input; f_b input; R_nb_err input; u output size=[3,1]; R_nb_stim input; b_stim input
function u = fcn(w_ib,f_b_dot,  f_b, R_nb_err,R_nb_stim, b_stim)

% hp: b_err = b_true - b_stim = 0 - b_stim = -b_stim

Skew_of_w = skew(w_ib);
Skew_of_b = skew(-b_stim);

u = (R_nb_err * f_b_dot) + (R_nb_err * Skew_of_w * f_b) - (R_nb_stim * Skew_of_b * f_b);

end

== matlab function Copy_of_model/error/MATLAB Function ==
  data: u input; y1 output; y2 output; y3 output; y4 output
function [y1,y2,y3,y4] = fcn(u)

y1 = u(1:3,1);
y2 = u(4,1);
y3 = u(5:7,1);
y4 = u(8:10,1);

end

== matlab function Copy_of_model/Kalman - Bucy Filter/C matrix ==
  data: C output; C_dx input
function C = Cfunc(C_dx)

   row = size(C_dx,1); 

   C1 = zeros(row,6);

 C = [2*C_dx C1];
 
 
end

== matlab function Copy_of_model/Attitude Observer/from body to NED frame ==
  data: m_b_mag input; t input; R_bn input; m_n_mag output
function m_n_mag = b2n(m_b_mag, t, R_bn)

% m_n_mag and m_b_mag are 3x1

% if t==0
%     R_bn = eye(3);
% end

m_n_mag = R_bn * m_b_mag;

== matlab function Copy_of_model/Attitude Observer/matrixInverse ==
  data: A input; AInv output
function AInv  = matrixInverse(A)

% AInv = inv(A);

% inverse by singular value decomposition


[n,m] = size(A);

% % % U = zeros(n,n);
% % % V = zeros(n,n);
% % % S = zeros(n,n);

[U,S,V] = svd(A);

pos = 0;

% % % maximun admissible condition number
csi = 10^3;

for i=n:-1:1
    if( S(1,1)/S(i,i) > csi)
        S(i,i) = 0;
        pos = i; % keeps the last eliminated singular value
    end
end

tempS = S(1:pos-1,1:pos-1); %take the non-zero set
tempS = inv(tempS);
S(1:pos-1,1:pos-1) = tempS(1:pos-1,1:pos-1); % now S is the inverse matrix
AInv = V * S * U';

end

== matlab function Copy_of_model/Mechanisation/from angular velocity to euler angles ==
  data: w_ib input; phi input; theta input; phi_dot output; theta_dot output; psi_dot output
function [phi_dot, theta_dot, psi_dot] = w2doteuler(w_ib, phi, theta)


D = zeros(3,3);
D(1,1) = 1;
D(1,2) = sin(phi)*tan(theta);
D(1,3) = cos(phi)*tan(theta);

D(2,2) = cos(phi);
D(2,3) = -sin(phi);

D(3,2) = sin(phi)/cos(theta);
D(3,3) = cos(phi)/cos(theta); 


% D = [ 1    sin(phi)*tan(theta)     cos(phi)*tan(theta);
%       0        cos(phi)                - sin(phi);
%       0    sin(phi)/cos(theta)     cos(phi)/cos(theta)]; 

phi_dot = D(1,:) * w_ib;
theta_dot = D(2,:) * w_ib;
psi_dot = D(3,:) * w_ib;

end

== matlab function Copy_of_model/Mechanisation/MATLAB Function ==
  data: phi input; R output; theta input; psi input
function R = eul2R(phi, theta, psi)

angles = [phi theta psi];

R = eul2rotm(angles,'ZYX');

end

== matlab function Copy_of_model/Mechanisation/MATLAB Function1 ==
  data: u input; y output
function y = fcn(u)

y = norm(u);

== matlab function Copy_of_model/Mechanisation/mechanisation ==
  data: f_b input; v_n_dot output; R_nb input
function v_n_dot  = mechanisation(f_b, R_nb)

g_n = [0.1 0.1 0.1]';   % gravity compensated

v_n_dot = R_nb * f_b + g_n;

end

== matlab function Copy_of_model/Attitude Observer/MATLAB Function ==
  data: u input; y output
function y = fcn(u)

% ckecking if norm == 1

y = norm(u,2);

== matlab function Copy_of_model/Attitude Observer/MATLAB Function3 ==
  data: u input; y output
function y = fcn(u)

y = norm(u);

== matlab function Copy_of_model/Algebraic Transformation/algebraic transform solution ==
  data: C_dx input; x_at output; delta input size=[5,1]
function x_at = solAT(C_dx, delta)

% inverse

pC_dx = pinv(C_dx);

x_at = pC_dx * (delta / 2);


% % % % [n,m] = size(C_dx);
% % % % 
% % % % % U = zeros(n,n);
% % % % % V = zeros(n,n);
% % % % % S = zeros(n,n);
% % % % 
% % % % [U,S,V] = svd(C_dx);
% % % % 
% % % % pos = 0;
% % % % 
% % % % % maximun admissible condition number
% % % % csi = 10^3;
% % % % 
% % % % for i=m:-1:1
% % % %     if( S(1,1)/S(i,i) > csi)
% % % %         S(i,i) = 0;
% % % %         pos = i; % keeps the last eliminated singular value
% % % %     end
% % % % end
% % % % 
% % % % % rebuild C_dx matrix
% % % % C_dx = U * S * V';
% % % % 
% % % % % % tempS = S(1:pos-1,1:pos-1); %take the non-zero set
% % % % % % tempS = inv(tempS);
% % % % % % S(1:pos-1,1:pos-1) = tempS(1:pos-1,1:pos-1); % now S is the inverse matrix
% % % % % % AInv = V * S * U';
% % % % 
% % % % 
% % % % % this solution is described in the Appendix
% % % % % and it is true only for m >= 5




end

== matlab function Copy_of_model/Gain computation/Discrete Riccati Equation/MATLAB Function ==
  data: A input; y output; C input; Q input; R input; P input; k output
function [y,k] = fcn(A,C,Q,R,P)

% %%% good inversion
% 
% temp = C*P*C' + R;
% 
% [n,m] = size(temp);
% 
% [U,S,V] = svd(temp);
% 
% pos = 0;
% 
% % maximun admissible condition number
% csi = 10^3;
% 
% for i=n:-1:1
%     if( S(1,1)/S(i,i) > csi)
%         S(i,i) = 0;
%         pos = i; % keeps the last eliminated singular value
%     end
% end
% 
% tempNZ = S(1:pos-1,1:pos-1); %take the non-zero set
% tempI = inv(tempNZ);
% S(1:pos-1,1:pos-1) = tempI(1:pos-1,1:pos-1); % now S is the inverse matrix
% new_inv = V * S * U';
 

%%% Discrete Riccati Equation



% y = Q + A'*P*A - A'*P*C'*(new_inv)*C*P*A;
y = Q + A'*P*A - A'*P*C'*(inv(C*P*C' + R))*C*P*A;
 

%%% Gain Matrix
% % 
% % k = new_inv*C*P*A;
% k = inv(C*P*C' + R)*C*P*A;

k = A'*P*C'*(inv(C*P*C' + R));

== matlab function Copy_of_model/Translational Motion Observer/MATLAB Function1 ==
  data: K input; K1 output; K2 output; K3 output; K4 output
function [K1,K2,K3,K4] = divK(K)

 K1 = K(1:3,:); 
 K2 = K(4,:);
 K3 = K(5:7,:);
 K4 = K(8:10,:);
 
end

== matlab function Copy_of_model/Translational Motion Observer/EPS ==
  data: K4 input; epsilon_dot output; K_p input; sigma input; J_stim input; f_b_imu input; corr input
function epsilon_dot = accel(K4,K_p, sigma, J_stim, f_b_imu, corr)

epsilon_dot   = -sigma * K_p * J_stim * f_b_imu + K4 * (corr); % eq 17

end

== matlab function Copy_of_model/Translational Motion Observer/ACC ==
  data: epsilon input; R_nb_stim input; f_n_stim output; f_b_imu input
function f_n_stim = fcn(epsilon,R_nb_stim, f_b_imu)

f_n_stim = R_nb_stim * f_b_imu + epsilon ;

end

== matlab function Copy_of_model/Translational Motion Observer/VEL ==
  data: K3 input; f_n_stim input; v_n_dot_stim output; corr input
function v_n_dot_stim = fcn(K3,f_n_stim, corr)

g_n = [0.1;0.1;0.1];

v_n_dot_stim = f_n_stim + g_n + K3*(corr);

== matlab function Copy_of_model/Translational Motion Observer/POSITION ==
  data: K1 input; v_n_stim input; p_n_delta_dot_stim output; corr input
function p_n_delta_dot_stim  = fcn(K1,v_n_stim,corr)

p_n_delta_dot_stim = v_n_stim + K1 * (corr);       % eq 14

end

== matlab function Copy_of_model/Translational Motion Observer/BETA ==
  data: K2 input; beta_dot_stim output; corr input
function beta_dot_stim = fcn(K2,corr)

beta_dot_stim = K2 * (corr);

== matlab function Copy_of_model/Translational Motion Observer/MATLAB Function2 ==
  data: u2 input; u1 input; new_x_stim output size=[4,1]
function new_x_stim = fcn(u2,u1)

new_x_stim = zeros(4,1);

new_x_stim(1:3,1) = u1;
new_x_stim(4,1) = u2;

end

== matlab function Copy_of_model/Translational Motion Observer/corr ==
  data: delta input; y output size=[5,1]; C_dx input; x_stim input size=[4,1]
function y = fcn(delta, C_dx, x_stim)

% delta and C_dx_x comes from algebraic transformation
% the first x_stim too, then by NLO

y = (delta - C_dx*x_stim) ;

== matlab function Copy_of_model/Gain computation/Discrete Riccati Equation/MATLAB Function1 ==
  data: u input; y output
function y = fcn(u)

y = norm(u,2);

== matlab function Copy_of_model/Gain computation/Discrete Riccati Equation/MATLAB Function2 ==
  data: u input; y output
function y = fcn(u)

y = norm(u,inf);

== matlab function Copy_of_model/Gain computation/Discrete Riccati Equation/MATLAB Function5 ==
  data: y output
function y = fcn()

% gain computed by dare

% y =   [      0         0         0         0         0;
%          0         0         0         0         0;
%          0         0         0         0         0;
%          0         0         0         0         0;
%     0.0041   -0.0073    0.0034   -0.0061   -0.0027;
%     0.0019   -0.0042    0.0025   -0.0039   -0.0014;
%     0.0064    0.0627   -0.0137   -0.0051    0.0087;
%          0         0         0         0         0;
%          0         0         0         0         0;
%          0         0         0         0         0];


%    y = [     0         0         0         0         0;
%              0         0         0         0         0;
%              0         0         0         0         0;
%              0         0         0         0         0;
%         0.0041   -0.0073    0.0034   -0.0062   -0.0026;
%         0.0019   -0.0042    0.0025   -0.0039   -0.0014;
%         0.0060    0.0636   -0.0139   -0.0043    0.0085;
%              0         0         0         0         0;
%              0         0         0         0         0;
%              0         0         0         0         0];




y = 0.0000001*[338.0836 -251.3072 -528.1877 -619.4670 -399.7782;
 -535.8536   27.3842  454.0360 -710.6385   30.9063;
  191.9185  938.7820 -163.0274 -207.9268  109.7480;
  737.8810  -69.3387  656.6684 -138.8543   15.1638;
    0.0037   -0.0066    0.0031   -0.0056   -0.0027;
    0.0018   -0.0039    0.0024   -0.0036   -0.0015;
    0.0076    0.0605   -0.0128   -0.0068    0.0087;
    0.0000   -0.0000    0.0000   -0.0000   -0.0000;
    0.0000   -0.0000    0.0000   -0.0000   -0.0000;
    0.0000    0.0000   -0.0000   -0.0000    0.0000];
